simulink model "plant_VV_l"  (R2023a)
settings: Solver=FixedStepAuto  StartTime=0.0  StopTime=10.0  FixedStep=0.01  RelTol=1e-3
undefined symbols (not defined in the file or in its folder): sys
libraries: simulink_extras x2
settings Model: Creator=timme  LastModifiedBy=timme
settings OptimizationCC: BlockReduction=off  DefaultParameterBehavior=Inlined  BufferReuse=off

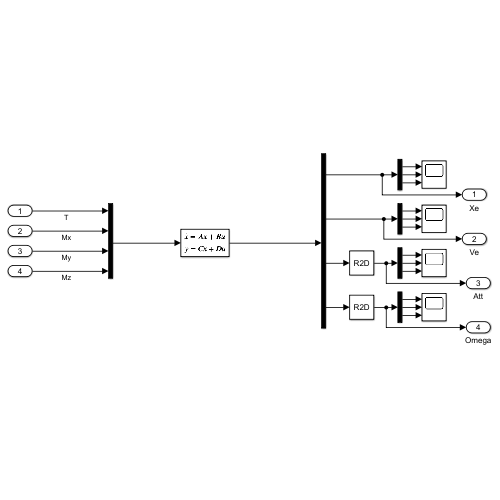
[thumbnail: Simulink's stored preview of the top-level diagram]
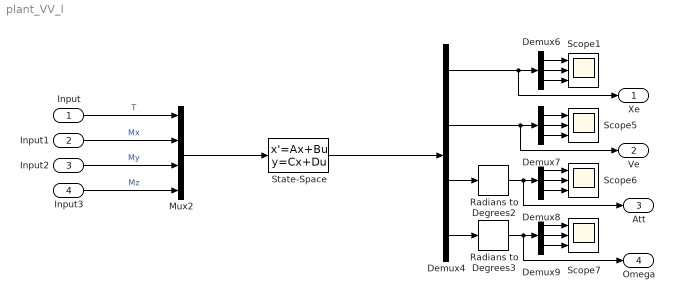
== system plant_VV_l ==
  Input : Inport
  Input1 : Inport  Port=2
  Input2 : Inport  Port=3
  Input3 : Inport  Port=4
  Demux4 : Demux  Outputs=[3 3 3 3]
  Demux{6..9} (4 alike) : Demux  Outputs=3
  Mux2 : Mux
  Radians to Degrees2 : simulink_extras/Transformations/Radians to Degrees
  Radians to Degrees3 : simulink_extras/Transformations/Radians to Degrees
  Scope{1,5..7} (4 alike) : Scope  NumInputPorts=3
  State-Space : StateSpace  A=sys.A  B=sys.B  C=sys.C  D=sys.D  InitialCondition=0
  Xe : Outport
  Ve : Outport  Port=2
  Att : Outport  Port=3
  Omega : Outport  Port=4
  wires:
  Input1/1 -> Mux2/2  "Mx"
  Input/1 -> Mux2/1  "T"
  Demux7/2 -> Scope5/2
  Demux4/2 -> Ve/1, Demux7/1
  Demux7/3 -> Scope5/3
  Demux6/2 -> Scope1/2
  Radians to Degrees3/1 -> Omega/1, Demux9/1
  Demux9/1 -> Scope7/1
  State-Space/1 -> Demux4/1
  Demux9/2 -> Scope7/2
  Demux8/1 -> Scope6/1
  Demux4/3 -> Radians to Degrees2/1
  Demux4/4 -> Radians to Degrees3/1
  Demux6/3 -> Scope1/3
  Demux7/1 -> Scope5/1
  Radians to Degrees2/1 -> Att/1, Demux8/1
  Demux6/1 -> Scope1/1
  Demux9/3 -> Scope7/3
  Demux4/1 -> Xe/1, Demux6/1
  Demux8/3 -> Scope6/3
  Demux8/2 -> Scope6/2
  Mux2/1 -> State-Space/1
  Input2/1 -> Mux2/3  "My"
  Input3/1 -> Mux2/4  "Mz"
